simulink model "Example_Sending_UDP_Video_In_Normal_Mode"  (R2016a)
settings: configuration reference "AR_Drone_ConfigSet_NOEXT" (kept outside this file)
libraries: AR_Drone_Video x1, AR_Drone_Networking x1, dspnetwork x1, AR_Drone_Video_Processing x1
settings Model: DataDictionary=ArDroneDataDictionary.sldd  Creator=sannem  LastModifiedBy=sannem
settings ConfigSetRef: DDName=ArDroneDataDictionary.sldd

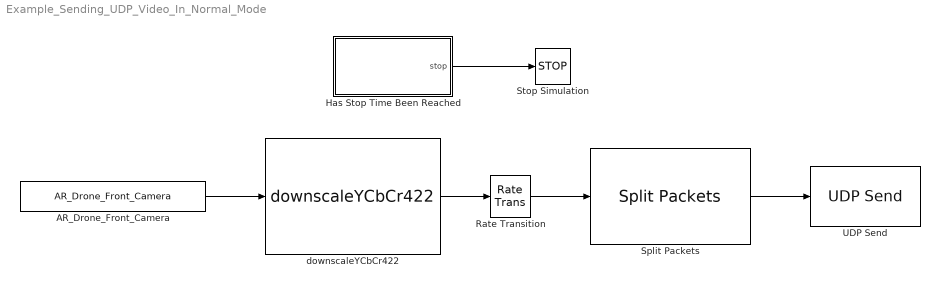
== system Example_Sending_UDP_Video_In_Normal_Mode ==
  AR_Drone_Front_Camera : AR_Drone_Video/AR_Drone_Front_Camera  SFunctionSpec=videoGrabImage1(uint8 y1[1843200])  SampleTime=0.1  ShowSpec=off
  Has Stop Time Been Reached : MATLAB Function  TreatAsAtomicUnit=on  SystemSampleTime=sampleTime  mask{stopTime=100, sampleTime=1/10}
      mask prompts: stopTime "Stop time [s]"; sampleTime "Sample time [s]"
      mask help: This block will keep track of the run time of a model. The default output is "0" with the output changing to "1" if the run time exceeds the user specified stop time.
  Rate Transition : RateTransition  OutPortSampleTime=1/100
  Split Packets : AR_Drone_Networking/Split Packets  bytesPerPacket=15000
  Stop Simulation : Stop
  UDP Send : dspnetwork/UDP Send  remoteURL='192.168.1.2'  remotePort=24000  localURL='0.0.0.0'  localPortSource=Automatically determine  localPort=-1  sampletime=-1  blockPlatform=LINUX  separateLengthPort=0  mask(UDP Send){}
  downscaleYCbCr422 : AR_Drone_Video_Processing/downscaleYCbCr422  width=1280  height=720  downScaleFactor=5
  wires:
  AR_Drone_Front_Camera/1 -> downscaleYCbCr422/1
  Rate Transition/1 -> Split Packets/1
  downscaleYCbCr422/1 -> Rate Transition/1
  Split Packets/1 -> UDP Send/1
  Has Stop Time Been Reached/1(stop) -> Stop Simulation/1

== matlab function Example_Sending_UDP_Video_In_Normal_Mode/Has Stop Time Been Reached ==
  data: stop output; stopTime parameter; sampleTime parameter
function stop = stopTimeReached(stopTime,sampleTime)
%#codegen

% persistent variable which keeps track of the total run time
persistent runTime
if isempty(runTime)
    runTime = sampleTime
else
    runTime = runTime + sampleTime;
end

stop = 0;
% verify whether the stop time is reached
if runTime > stopTime
    stop = 1;
end
